simulink model "sampleModel106"  (R2022a)
settings: Solver=VariableStepAuto  StartTime=0.0  StopTime=10.0  RelTol=1e-3
undefined symbols (not defined in the file): DiscIntNeverNeededParam, magnitude, Newton, Raphson
libraries: simulink x379, slpidlib x89
(part 15 of 16)

== system sampleModel106/cfblk86/cfblk11/cfblk7/cfblk7 ==
  cfblk1 : Inport
  cfblk13 : Inport  Port=2
  cfblk14 : Inport  Port=3
  cfblk10 : Assignment  DiagnosticForDimensions=Warning  IndexOptions=Index vector (dialog)  Indices=1  OutputSizes=1
  cfblk11 : Constant  Value=[926177037.249093]  SampleTime=1
  cfblk12 : Constant  Value=[191997706.928792]  SampleTime=1
  cfblk15 : Delay
  cfblk16 : Delay
  cfblk3 : slpidlib/PID Controller (2DOF)  Controller=PID  Form=Parallel  TimeDomain=Discrete-time  UseExternalTs=off  SampleTime=-1  IntegratorMethod=Forward Euler  FilterMethod=Forward Euler  ControllerParametersSource=internal  P=1  I=1  UseKiTs=off  D=0  N=100  UseFilter=on  b=1  c=1  TunerSelectOption=Transfer Function Based (PID Tuner App)  InitialConditionSource=internal  InitialConditionForIntegrator=0  InitialConditionForFilter=0  DifferentiatorICPrevScaledInput=0  ExternalReset=none  TrackingMode=off  Kt=1  LimitOutput=off  SatLimitsSource=internal  UpperSaturationLimit=inf  LowerSaturationLimit=-inf  LinearizeAsGain=off  AntiWindupMode=none  Kb=1  POutMin=[]  POutMax=[]  IOutMin=[]  IOutMax=[]  DOutMin=[]  DOutMax=[]  NOutMin=[]  NOutMax=[]  bOutMin=[]  bOutMax=[]  cOutMin=[]  cOutMax=[]  SumOutMin=[]  SumOutMax=[]  SaturationOutMin=[]  SaturationOutMax=[]  PParamMin=[]  PParamMax=[]  IParamMin=[]  IParamMax=[]  DParamMin=[]  DParamMax=[]  NParamMin=[]  NParamMax=[]  bParamMin=[]  bParamMax=[]  cParamMin=[]  cParamMax=[]  KbParamMin=[]  KbParamMax=[]  KtParamMin=[]  KtParamMax=[]  KbOutMin=[]  KbOutMax=[]  KtOutMin=[]  KtOutMax=[]  IntegratorOutMin=[]  IntegratorOutMax=[]  FilterOutMin=[]  FilterOutMax=[]  SumI1OutMin=[]  SumI1OutMax=[]  SumI2OutMin=[]  SumI2OutMax=[]  SumI3OutMin=[]  SumI3OutMax=[]  SumI4OutMin=[]  SumI4OutMax=[]  SumDOutMin=[]  SumDOutMax=[]  Sum1OutMin=[]  Sum1OutMax=[]  Sum2OutMin=[]  Sum2OutMax=[]  Sum3OutMin=[]  Sum3OutMax=[]  DifferentiatorOutMin=[]  DifferentiatorOutMax=[]  FilterDiffOutCoefMin=[]  FilterDiffOutCoefMax=[]  ReciprocalOutMin=[]  ReciprocalOutMax=[]  SumDenOutMin=[]  SumDenOutMax=[]  SumNumOutMin=[]  SumNumOutMax=[]  DivideOutMin=[]  DivideOutMax=[]  UdiffTsProdOutMin=[]  UdiffTsProdOutMax=[]  NTsProdOutMin=[]  NTsProdOutMax=[]  UintegralTsProdOutMin=[]  UintegralTsProdOutMax=[]  UngainTsProdOutMin=[]  UngainTsProdOutMax=[]  IntegratorContinuousStateAttributes=''  IntegratorStateMustResolveToSignalObject=off  IntegratorRTWStateStorageClass=Auto  FilterContinuousStateAttributes=''  FilterStateMustResolveToSignalObject=off  FilterRTWStateStorageClass=Auto  ParallelPVariant=InternalParameters  IdealPVariant=Disabled  IVariant=InternalParameters  DVariant=InternalParameters  bVariant=InternalParameters  cVariant=InternalParameters  IntegratorVariant=Discrete  SatVariant=Disabled  AWVariant=Passthrough  PCopyVariant=Disabled  TRVariant=Disabled  FdbkBlocksVariant=Forward  IdealPFdbkVariant=Disabled  SatFdbkVariant=Disabled  DerivativeFilterVariant=ForwardEulerFilter  NVariant=InternalParameters  NCopyVariant=Disabled  FilterICVariant=InternalICsFilter  IntegratorICVariant=InternalICs  ExternalResetVariant=Disabled  TRSumVariant=Passthrough  SumFdbkVariant=Disabled  SumVariant=Sum_PID  TsampFilterVariant=InternalTs  TsampNgainVariant=Passthrough  TsampIntegralVariant=Passthrough  ExternalSaturationOutDataTypeStr=Inherit: Same as second input
      settings: SourceProductBaseCode=SL
  cfblk4 : simulink/Discrete/Transfer Fcn Real Zero  ZeroZ=0.75  ICPrevInput=0.0  DoSatur=off
      settings: SourceProductBaseCode=SL
  cfblk5 : Signum
  cfblk6 : Product
  cfblk7 : Sum  Inputs=-+
  cfblk8 : Sum  Inputs=|++
  cfblk9 : PermuteDimensions
  cfblk2 : Outport
  wires:
  cfblk1/1 -> cfblk6/1
  cfblk14/1 -> cfblk5/1
  cfblk12/1 -> cfblk8/1
  cfblk3/1 -> cfblk9/1
  cfblk11/1 -> cfblk6/2
  cfblk8/1 -> cfblk3/2, cfblk7/2
  cfblk6/1 -> cfblk2/1
  cfblk7/1 -> cfblk10/1
  cfblk4/1 -> cfblk10/2
  cfblk5/1 -> cfblk8/2
  cfblk13/1 -> cfblk7/1
  cfblk9/1 -> cfblk15/1
  cfblk15/1 -> cfblk3/1
  cfblk10/1 -> cfblk16/1
  cfblk16/1 -> cfblk4/1

== system sampleModel106/cfblk86/cfblk11/cfblk7/cfblk8 ==
  cfblk1 : Inport
  cfblk16 : Inport  Port=2
  cfblk10 : UnaryMinus
  cfblk11 : UnaryMinus
  cfblk12 : Constant  Value=[368440293.841524]  SampleTime=1
  cfblk13 : Constant  Value=[930895856.774542]  SampleTime=1
  cfblk14 : Constant  Value=[721603009.060118]  SampleTime=1
  cfblk15 : Constant  Value=[-108594991.261578]  SampleTime=1
  cfblk3 : Delay  ShowEnablePort=on
      settings: InputPortMap=u0,e6
  cfblk4 : simulink/Discrete/Tapped Delay  vinit=0.0  samptime=-1  NumDelays=1  DelayOrder=Oldest  includeCurrent=off
  cfblk5 : Sqrt  Operator=rSqrt  AlgorithmType=Newton-Raphson
  cfblk6 : Sum  Inputs=|++
  cfblk7 : Sum  Inputs=+
  cfblk8 : Squeeze
  cfblk9 : UnaryMinus
  cfblk2 : Outport
  wires:
  cfblk9/1 -> cfblk6/1
  cfblk3/1 -> cfblk5/1
  cfblk12/1 -> cfblk7/1
  cfblk15/1 -> cfblk2/1
  cfblk13/1 -> cfblk8/1
  cfblk8/1 -> cfblk6/2
  cfblk10/1 -> cfblk9/1
  cfblk16/1 -> cfblk10/1
  cfblk6/1 -> cfblk4/1
  cfblk1/1 -> cfblk11/1
  cfblk14/1 -> cfblk3/1
  cfblk7/1 -> cfblk3/2

== system sampleModel106/cfblk86/cfblk11/cfblk8/cfblk11 ==
  cfblk1 : Inport
  cfblk7 : Inport  Port=2
  cfblk3 : UnitDelay  SampleTime=-1  HasFrameUpgradeWarning=on
  cfblk4 : Constant  Value=[595381109.749089]  SampleTime=1
  cfblk5 : Constant  Value=[-747588408.733182]  SampleTime=1
  cfblk6 : Constant  Value=[-697953412.486928]  SampleTime=1
  cfblk2 : Outport
  wires:
  cfblk3/1 -> cfblk2/1
  cfblk1/1 -> cfblk3/1

== system sampleModel106/cfblk86/cfblk11/cfblk8/cfblk12 ==
  cfblk1 : Inport
  cfblk9 : Inport  Port=2
  cfblk10 : Delay
  cfblk11 : Delay
  cfblk3 : simulink/Discrete/Tapped Delay  vinit=0.0  samptime=-1  NumDelays=1  DelayOrder=Oldest  includeCurrent=off
  cfblk4 : PermuteDimensions
  cfblk5 : Math  Operator=transpose
  cfblk6 : Product  Inputs=**
  cfblk7 : DotProduct  OutDataTypeStr=Inherit: Inherit via internal rule
  cfblk8 : Constant  Value=[62268794.825662]  SampleTime=1
  cfblk2 : Outport
  wires:
  cfblk9/1 -> cfblk5/1
  cfblk7/1 -> cfblk3/1
  cfblk1/1 -> cfblk7/2
  cfblk4/1 -> cfblk6/1
  cfblk5/1 -> cfblk6/2
  cfblk8/1 -> cfblk2/1
  cfblk3/1 -> cfblk10/1
  cfblk10/1 -> cfblk7/1
  cfblk6/1 -> cfblk11/1
  cfblk11/1 -> cfblk4/1

== system sampleModel106/cfblk86/cfblk12/cfblk10/cfblk17 ==
  cfblk1 : Inport
  cfblk14 : Inport  Port=2
  Action Port : ActionPort  ActionPortLabel=if(u1 >= 0)
  cfblk10 : Product
  cfblk11 : Polyval  Coefs=[ +2.081618890e-019, -1.441693666e-014, +4.719686976e-010, -8.536869453e-006, +1.621573104e-001, -8.087801117e+001 ]
  cfblk12 : Sum  Inputs=-+
  cfblk13 : Constant  Value=[-942667236.910500]  SampleTime=1
  cfblk16 : Delay
  cfblk17 : Delay
  cfblk3 : DiscreteFir
  cfblk4 : slpidlib/PID Controller (2DOF)  Controller=PID  Form=Parallel  TimeDomain=Discrete-time  UseExternalTs=off  SampleTime=-1  IntegratorMethod=Forward Euler  FilterMethod=Forward Euler  ControllerParametersSource=internal  P=1  I=1  UseKiTs=off  D=0  N=100  UseFilter=on  b=1  c=1  TunerSelectOption=Transfer Function Based (PID Tuner App)  InitialConditionSource=internal  InitialConditionForIntegrator=0  InitialConditionForFilter=0  DifferentiatorICPrevScaledInput=0  ExternalReset=none  TrackingMode=off  Kt=1  LimitOutput=off  SatLimitsSource=internal  UpperSaturationLimit=inf  LowerSaturationLimit=-inf  LinearizeAsGain=off  AntiWindupMode=none  Kb=1  POutMin=[]  POutMax=[]  IOutMin=[]  IOutMax=[]  DOutMin=[]  DOutMax=[]  NOutMin=[]  NOutMax=[]  bOutMin=[]  bOutMax=[]  cOutMin=[]  cOutMax=[]  SumOutMin=[]  SumOutMax=[]  SaturationOutMin=[]  SaturationOutMax=[]  PParamMin=[]  PParamMax=[]  IParamMin=[]  IParamMax=[]  DParamMin=[]  DParamMax=[]  NParamMin=[]  NParamMax=[]  bParamMin=[]  bParamMax=[]  cParamMin=[]  cParamMax=[]  KbParamMin=[]  KbParamMax=[]  KtParamMin=[]  KtParamMax=[]  KbOutMin=[]  KbOutMax=[]  KtOutMin=[]  KtOutMax=[]  IntegratorOutMin=[]  IntegratorOutMax=[]  FilterOutMin=[]  FilterOutMax=[]  SumI1OutMin=[]  SumI1OutMax=[]  SumI2OutMin=[]  SumI2OutMax=[]  SumI3OutMin=[]  SumI3OutMax=[]  SumI4OutMin=[]  SumI4OutMax=[]  SumDOutMin=[]  SumDOutMax=[]  Sum1OutMin=[]  Sum1OutMax=[]  Sum2OutMin=[]  Sum2OutMax=[]  Sum3OutMin=[]  Sum3OutMax=[]  DifferentiatorOutMin=[]  DifferentiatorOutMax=[]  FilterDiffOutCoefMin=[]  FilterDiffOutCoefMax=[]  ReciprocalOutMin=[]  ReciprocalOutMax=[]  SumDenOutMin=[]  SumDenOutMax=[]  SumNumOutMin=[]  SumNumOutMax=[]  DivideOutMin=[]  DivideOutMax=[]  UdiffTsProdOutMin=[]  UdiffTsProdOutMax=[]  NTsProdOutMin=[]  NTsProdOutMax=[]  UintegralTsProdOutMin=[]  UintegralTsProdOutMax=[]  UngainTsProdOutMin=[]  UngainTsProdOutMax=[]  IntegratorContinuousStateAttributes=''  IntegratorStateMustResolveToSignalObject=off  IntegratorRTWStateStorageClass=Auto  FilterContinuousStateAttributes=''  FilterStateMustResolveToSignalObject=off  FilterRTWStateStorageClass=Auto  ParallelPVariant=InternalParameters  IdealPVariant=Disabled  IVariant=InternalParameters  DVariant=InternalParameters  bVariant=InternalParameters  cVariant=InternalParameters  IntegratorVariant=Discrete  SatVariant=Disabled  AWVariant=Passthrough  PCopyVariant=Disabled  TRVariant=Disabled  FdbkBlocksVariant=Forward  IdealPFdbkVariant=Disabled  SatFdbkVariant=Disabled  DerivativeFilterVariant=ForwardEulerFilter  NVariant=InternalParameters  NCopyVariant=Disabled  FilterICVariant=InternalICsFilter  IntegratorICVariant=InternalICs  ExternalResetVariant=Disabled  TRSumVariant=Passthrough  SumFdbkVariant=Disabled  SumVariant=Sum_PID  TsampFilterVariant=InternalTs  TsampNgainVariant=Passthrough  TsampIntegralVariant=Passthrough  ExternalSaturationOutDataTypeStr=Inherit: Same as second input
      settings: SourceProductBaseCode=SL
  cfblk5 : DiscreteIntegrator  SampleTime=-1  ICPrevOutput=DiscIntNeverNeededParam  ICPrevScaledInput=DiscIntNeverNeededParam
  cfblk6 : Sqrt  Operator=rSqrt  AlgorithmType=Newton-Raphson
  cfblk7 : Sin  TimeSource=Use external signal  SampleTime=0
  cfblk8 : Sum  Inputs=--
  cfblk9 : Rounding
  cfblk2 : Outport
  cfblk15 : Outport  Port=2
  wires:
  cfblk6/1 -> cfblk12/1
  cfblk14/1 -> cfblk6/1
  cfblk11/1 -> cfblk12/2, cfblk10/2
  cfblk9/1 -> cfblk10/1
  cfblk13/1 -> cfblk3/1
  cfblk12/1 -> cfblk8/1, cfblk17/1
  cfblk3/1 -> cfblk15/1, cfblk5/1
  cfblk8/1 -> cfblk9/1
  cfblk4/1 -> cfblk11/1
  cfblk10/1 -> cfblk7/1
  cfblk5/1 -> cfblk2/1
  cfblk1/1 -> cfblk4/1
  cfblk7/1 -> cfblk16/1
  cfblk16/1 -> cfblk8/2
  cfblk17/1 -> cfblk4/2

== system sampleModel106/cfblk86/cfblk12/cfblk10/cfblk18 ==
  cfblk1 : Inport
  cfblk10 : Inport  Port=2
  cfblk11 : Inport  Port=3
  Action Port : ActionPort  ActionPortLabel=else
  cfblk3 : Delay  DelayLengthSource=Input port
      settings: InputPortMap=u0,p1
  cfblk4 : simulink/Discrete/Tapped Delay  vinit=0.0  samptime=-1  NumDelays=1  DelayOrder=Oldest  includeCurrent=off
  cfblk5 : DotProduct  OutDataTypeStr=Inherit: Inherit via internal rule
  cfblk6 : Squeeze
  cfblk7 : Constant  Value=[600315880.016551]  SampleTime=1
  cfblk8 : Constant  Value=[-855675458.268582]  SampleTime=1
  cfblk9 : Constant  Value=[266092827.562817]  SampleTime=1
  cfblk2 : Outport
  cfblk12 : Outport  Port=2
  wires:
  cfblk3/1 -> cfblk5/1
  cfblk9/1 -> cfblk5/2
  cfblk10/1 -> cfblk4/1
  cfblk6/1 -> cfblk12/1
  cfblk8/1 -> cfblk3/1
  cfblk5/1 -> cfblk2/1
  cfblk1/1 -> cfblk3/2
  cfblk11/1 -> cfblk6/1

== system sampleModel106/cfblk86/cfblk12/cfblk11/cfblk10 ==
  cfblk1 : Inport
  cfblk11 : Inport  Port=2
  cfblk12 : Inport  Port=3
  cfblk13 : Inport  Port=4
  cfblk14 : Inport  Port=5
  cfblk10 : Constant  Value=[814482863.956402]  SampleTime=1
  cfblk3 : DiscreteStateSpace  SampleTime=-1
  cfblk4 : ComplexToRealImag
  cfblk5 : Gain  Gain=[-106543572.011716]
  cfblk6 : Signum
  cfblk7 : Abs  SaturateOnIntegerOverflow=off
  cfblk8 : Constant  Value=[-718916062.410219]  SampleTime=1
  cfblk9 : Constant  Value=[-797646911.590380]  SampleTime=1
  cfblk2 : Outport
  cfblk15 : Outport  Port=2
  wires:
  cfblk11/1 -> cfblk3/1
  cfblk13/1 -> cfblk15/1
  cfblk10/1 -> cfblk2/1
  cfblk4/1 -> cfblk5/1
  cfblk14/1 -> cfblk6/1
  cfblk3/1 -> cfblk4/1
  cfblk5/1 -> cfblk7/1

== system sampleModel106/cfblk86/cfblk12/cfblk11/cfblk11 ==
  cfblk1 : Inport
  cfblk10 : Inport  Port=2
  cfblk3 : simulink/Discrete/Transfer Fcn Real Zero  ZeroZ=0.75  ICPrevInput=0.0  DoSatur=off
      settings: SourceProductBaseCode=SL
  cfblk4 : UnitDelay  SampleTime=-1  HasFrameUpgradeWarning=on
  cfblk5 : Sum  Inputs=|++
  cfblk6 : PermuteDimensions
  cfblk7 : Gain  Gain=[693347693.453758]
  cfblk8 : Sum  Inputs=+
  cfblk9 : Gain  Gain=[980910987.680085]
  cfblk2 : Outport
  cfblk11 : Outport  Port=2
  cfblk12 : Outport  Port=3
  cfblk13 : Outport  Port=4
  wires:
  cfblk10/1 -> cfblk6/1, cfblk3/1
  cfblk9/1 -> cfblk11/1
  cfblk4/1 -> cfblk7/1
  cfblk1/1 -> cfblk8/1, cfblk2/1
  cfblk8/1 -> cfblk5/1, cfblk12/1
  cfblk5/1 -> cfblk9/1
  cfblk3/1 -> cfblk4/1
  cfblk6/1 -> cfblk5/2
  cfblk7/1 -> cfblk13/1

== system sampleModel106/cfblk86/cfblk12/cfblk11/cfblk12 ==
  cfblk1 : Inport
  cfblk13 : Inport  Port=2
  cfblk14 : Inport  Port=3
  cfblk10 : Gain  Gain=[-17064317.644250]
  cfblk11 : Abs  SaturateOnIntegerOverflow=off
  cfblk12 : Gain  Gain=[-145283411.917414]
  cfblk{16..19} (4 alike) : Delay
  cfblk3 : simulink/Discrete/Tapped Delay  vinit=0.0  samptime=-1  NumDelays=1  DelayOrder=Oldest  includeCurrent=off
  cfblk4 : Delay  ShowEnablePort=on
      settings: InputPortMap=u0,e6
  cfblk5 : Delay  DelayLengthSource=Input port
      settings: InputPortMap=u0,p1
  cfblk6 : slpidlib/PID Controller (2DOF)  Controller=PID  Form=Parallel  TimeDomain=Discrete-time  UseExternalTs=off  SampleTime=-1  IntegratorMethod=Forward Euler  FilterMethod=Forward Euler  ControllerParametersSource=internal  P=1  I=1  UseKiTs=off  D=0  N=100  UseFilter=on  b=1  c=1  TunerSelectOption=Transfer Function Based (PID Tuner App)  InitialConditionSource=internal  InitialConditionForIntegrator=0  InitialConditionForFilter=0  DifferentiatorICPrevScaledInput=0  ExternalReset=none  TrackingMode=off  Kt=1  LimitOutput=off  SatLimitsSource=internal  UpperSaturationLimit=inf  LowerSaturationLimit=-inf  LinearizeAsGain=off  AntiWindupMode=none  Kb=1  POutMin=[]  POutMax=[]  IOutMin=[]  IOutMax=[]  DOutMin=[]  DOutMax=[]  NOutMin=[]  NOutMax=[]  bOutMin=[]  bOutMax=[]  cOutMin=[]  cOutMax=[]  SumOutMin=[]  SumOutMax=[]  SaturationOutMin=[]  SaturationOutMax=[]  PParamMin=[]  PParamMax=[]  IParamMin=[]  IParamMax=[]  DParamMin=[]  DParamMax=[]  NParamMin=[]  NParamMax=[]  bParamMin=[]  bParamMax=[]  cParamMin=[]  cParamMax=[]  KbParamMin=[]  KbParamMax=[]  KtParamMin=[]  KtParamMax=[]  KbOutMin=[]  KbOutMax=[]  KtOutMin=[]  KtOutMax=[]  IntegratorOutMin=[]  IntegratorOutMax=[]  FilterOutMin=[]  FilterOutMax=[]  SumI1OutMin=[]  SumI1OutMax=[]  SumI2OutMin=[]  SumI2OutMax=[]  SumI3OutMin=[]  SumI3OutMax=[]  SumI4OutMin=[]  SumI4OutMax=[]  SumDOutMin=[]  SumDOutMax=[]  Sum1OutMin=[]  Sum1OutMax=[]  Sum2OutMin=[]  Sum2OutMax=[]  Sum3OutMin=[]  Sum3OutMax=[]  DifferentiatorOutMin=[]  DifferentiatorOutMax=[]  FilterDiffOutCoefMin=[]  FilterDiffOutCoefMax=[]  ReciprocalOutMin=[]  ReciprocalOutMax=[]  SumDenOutMin=[]  SumDenOutMax=[]  SumNumOutMin=[]  SumNumOutMax=[]  DivideOutMin=[]  DivideOutMax=[]  UdiffTsProdOutMin=[]  UdiffTsProdOutMax=[]  NTsProdOutMin=[]  NTsProdOutMax=[]  UintegralTsProdOutMin=[]  UintegralTsProdOutMax=[]  UngainTsProdOutMin=[]  UngainTsProdOutMax=[]  IntegratorContinuousStateAttributes=''  IntegratorStateMustResolveToSignalObject=off  IntegratorRTWStateStorageClass=Auto  FilterContinuousStateAttributes=''  FilterStateMustResolveToSignalObject=off  FilterRTWStateStorageClass=Auto  ParallelPVariant=InternalParameters  IdealPVariant=Disabled  IVariant=InternalParameters  DVariant=InternalParameters  bVariant=InternalParameters  cVariant=InternalParameters  IntegratorVariant=Discrete  SatVariant=Disabled  AWVariant=Passthrough  PCopyVariant=Disabled  TRVariant=Disabled  FdbkBlocksVariant=Forward  IdealPFdbkVariant=Disabled  SatFdbkVariant=Disabled  DerivativeFilterVariant=ForwardEulerFilter  NVariant=InternalParameters  NCopyVariant=Disabled  FilterICVariant=InternalICsFilter  IntegratorICVariant=InternalICs  ExternalResetVariant=Disabled  TRSumVariant=Passthrough  SumFdbkVariant=Disabled  SumVariant=Sum_PID  TsampFilterVariant=InternalTs  TsampNgainVariant=Passthrough  TsampIntegralVariant=Passthrough  ExternalSaturationOutDataTypeStr=Inherit: Same as second input
      settings: SourceProductBaseCode=SL
  cfblk7 : Sum  Inputs=|++
  cfblk8 : MinMax
  cfblk9 : Sqrt  Operator=rSqrt  AlgorithmType=Newton-Raphson
  cfblk2 : Outport
  cfblk15 : Outport  Port=2
  wires:
  cfblk1/1 -> cfblk15/1
  cfblk4/1 -> cfblk10/1
  cfblk3/1 -> cfblk6/1
  cfblk13/1 -> cfblk11/1
  cfblk12/1 -> cfblk6/2, cfblk5/1
  cfblk9/1 -> cfblk8/1, cfblk19/1
  cfblk11/1 -> cfblk12/1
  cfblk5/1 -> cfblk7/1
  cfblk6/1 -> cfblk2/1, cfblk16/1
  cfblk7/1 -> cfblk9/1
  cfblk14/1 -> cfblk4/2
  cfblk16/1 -> cfblk3/1
  cfblk10/1 -> cfblk17/1
  cfblk17/1 -> cfblk4/1
  cfblk8/1 -> cfblk18/1
  cfblk18/1 -> cfblk7/2
  cfblk19/1 -> cfblk5/2

== system sampleModel106/cfblk86/cfblk12/cfblk6/cfblk6 ==
  cfblk1 : Inport
  cfblk3 : simulink/Discrete/Transfer Fcn Lead or Lag  PoleZ=0.95  ZeroZ=0.75  ICPrevOutput=0.0  ICPrevInput=0.0  DoSatur=off
      settings: SourceProductBaseCode=SL
  cfblk4 : Reshape
  cfblk5 : Squeeze
  cfblk6 : Constant  Value=[-595129306.114251]  SampleTime=1
  cfblk7 : Constant  Value=[616259366.976854]  SampleTime=1
  cfblk8 : Constant  Value=[-570551448.739363]  SampleTime=1
  cfblk2 : Outport
  wires:
  cfblk7/1 -> cfblk3/1
  cfblk8/1 -> cfblk2/1
  cfblk6/1 -> cfblk5/1
  cfblk5/1 -> cfblk4/1

== system sampleModel106/cfblk86/cfblk12/cfblk6/cfblk7 ==
  cfblk1 : Inport
  cfblk7 : Inport  Port=2
  cfblk8 : Inport  Port=3
  cfblk12 : Delay
  cfblk3 : DiscreteTransferFcn
  cfblk4 : Assignment  DiagnosticForDimensions=Warning  IndexOptions=Index vector (dialog)  Indices=1  OutputSizes=1
  cfblk5 : Sqrt  Operator=rSqrt  AlgorithmType=Newton-Raphson
  cfblk6 : Constant  Value=[325301502.909390]  SampleTime=1
  cfblk2 : Outport
  cfblk9 : Outport  Port=2
  cfblk10 : Outport  Port=3
  cfblk11 : Outport  Port=4
  wires:
  cfblk6/1 -> cfblk2/1
  cfblk8/1 -> cfblk9/1
  cfblk1/1 -> cfblk10/1
  cfblk7/1 -> cfblk4/1
  cfblk3/1 -> cfblk5/1
  cfblk4/1 -> cfblk11/1, cfblk12/1
  cfblk5/1 -> cfblk4/2
  cfblk12/1 -> cfblk3/1

== system sampleModel106/cfblk86/cfblk12/cfblk6/cfblk8 ==
  cfblk1 : Inport
  cfblk10 : Delay
  cfblk3 : simulink/Discrete/Transfer Fcn First Order  PoleZ=0.95  ICPrevOutput=0.0  DoSatur=off
  cfblk4 : Product  Inputs=*
  cfblk5 : Rounding
  cfblk6 : Product  Inputs=*
  cfblk7 : Constant  Value=[387925012.139757]  SampleTime=1
  cfblk2 : Outport
  cfblk8 : Outport  Port=2
  cfblk9 : Outport  Port=3
  wires:
  cfblk4/1 -> cfblk5/1
  cfblk3/1 -> cfblk6/1
  cfblk5/1 -> cfblk8/1, cfblk2/1
  cfblk7/1 -> cfblk9/1
  cfblk1/1 -> cfblk4/1
  cfblk6/1 -> cfblk10/1
  cfblk10/1 -> cfblk3/1

== system sampleModel106/cfblk86/cfblk12/cfblk6/cfblk9 ==
  cfblk1 : Inport
  cfblk7 : Inport  Port=2
  cfblk8 : Inport  Port=3
  cfblk9 : Inport  Port=4
  cfblk3 : DiscreteTransferFcn
  cfblk4 : Bias  Bias=[399680849.594782]  SaturateOnIntegerOverflow=off
  cfblk5 : Constant  Value=[-667207257.082441]  SampleTime=1
  cfblk6 : Constant  Value=[329987459.255104]  SampleTime=1
  cfblk2 : Outport
  cfblk10 : Outport  Port=2
  wires:
  cfblk5/1 -> cfblk4/1
  cfblk6/1 -> cfblk10/1
  cfblk8/1 -> cfblk2/1
  cfblk1/1 -> cfblk3/1

== system sampleModel106/cfblk86/cfblk12/cfblk7/cfblk7 ==
  cfblk1 : Inport
  cfblk12 : Inport  Port=2
  cfblk13 : Inport  Port=3
  cfblk14 : Inport  Port=4
  cfblk10 : Constant  Value=[-241295018.099493]  SampleTime=1
  cfblk11 : Constant  Value=[926092452.295912]  SampleTime=1
  cfblk3 : DiscreteIntegrator  SampleTime=-1  ICPrevOutput=DiscIntNeverNeededParam  ICPrevScaledInput=DiscIntNeverNeededParam
  cfblk4 : Product  Inputs=*
  cfblk5 : simulink/Math Operations/MinMax Running Resettable  Function=min  vinit=0.0
  cfblk6 : Sum  Inputs=+-
  cfblk7 : Polyval  Coefs=[ +2.081618890e-019, -1.441693666e-014, +4.719686976e-010, -8.536869453e-006, +1.621573104e-001, -8.087801117e+001 ]
  cfblk8 : ComplexToRealImag
  cfblk9 : Constant  Value=[-944350246.390381]  SampleTime=1
  cfblk2 : Outport
  cfblk15 : Outport  Port=2
  cfblk16 : Outport  Port=3
  wires:
  cfblk11/1 -> cfblk16/1
  cfblk12/1 -> cfblk4/1
  cfblk8/1 -> cfblk15/1
  cfblk7/1 -> cfblk5/1
  cfblk4/1 -> cfblk5/2
  cfblk5/1 -> cfblk3/1
  cfblk1/1 -> cfblk7/1
  cfblk10/1 -> cfblk2/1
  cfblk9/1 -> cfblk8/1
  cfblk13/1 -> cfblk6/1
  cfblk8/2 -> cfblk6/2

== system sampleModel106/cfblk86/cfblk12/cfblk7/cfblk8 ==
  cfblk1 : Inport
  cfblk11 : Inport  Port=2
  cfblk10 : Constant  Value=[209927963.411676]  SampleTime=1
  cfblk12 : Delay
  cfblk3 : DiscreteFir
  cfblk4 : Delay
  cfblk5 : slpidlib/PID Controller  Controller=PID  Form=Parallel  TimeDomain=Discrete-time  UseExternalTs=off  SampleTime=-1  IntegratorMethod=Forward Euler  FilterMethod=Forward Euler  ControllerParametersSource=internal  P=1  I=1  UseKiTs=off  D=0  N=100  UseFilter=on  TunerSelectOption=Transfer Function Based (PID Tuner App)  InitialConditionSource=internal  InitialConditionForIntegrator=0  InitialConditionForFilter=0  DifferentiatorICPrevScaledInput=0  ExternalReset=none  TrackingMode=off  Kt=1  LimitOutput=off  SatLimitsSource=internal  UpperSaturationLimit=inf  LowerSaturationLimit=-inf  LinearizeAsGain=off  AntiWindupMode=none  Kb=1  POutMin=[]  POutMax=[]  IOutMin=[]  IOutMax=[]  DOutMin=[]  DOutMax=[]  NOutMin=[]  NOutMax=[]  SumOutMin=[]  SumOutMax=[]  SaturationOutMin=[]  SaturationOutMax=[]  PParamMin=[]  PParamMax=[]  IParamMin=[]  IParamMax=[]  DParamMin=[]  DParamMax=[]  NParamMin=[]  NParamMax=[]  KbParamMin=[]  KbParamMax=[]  KtParamMin=[]  KtParamMax=[]  KbOutMin=[]  KbOutMax=[]  KtOutMin=[]  KtOutMax=[]  IntegratorOutMin=[]  IntegratorOutMax=[]  FilterOutMin=[]  FilterOutMax=[]  SumI1OutMin=[]  SumI1OutMax=[]  SumI2OutMin=[]  SumI2OutMax=[]  SumI3OutMin=[]  SumI3OutMax=[]  SumI4OutMin=[]  SumI4OutMax=[]  SumDOutMin=[]  SumDOutMax=[]  DifferentiatorOutMin=[]  DifferentiatorOutMax=[]  FilterDiffOutCoefMin=[]  FilterDiffOutCoefMax=[]  ReciprocalOutMin=[]  ReciprocalOutMax=[]  SumDenOutMin=[]  SumDenOutMax=[]  SumNumOutMin=[]  SumNumOutMax=[]  DivideOutMin=[]  DivideOutMax=[]  UdiffTsProdOutMin=[]  UdiffTsProdOutMax=[]  NTsProdOutMin=[]  NTsProdOutMax=[]  UintegralTsProdOutMin=[]  UintegralTsProdOutMax=[]  UngainTsProdOutMin=[]  UngainTsProdOutMax=[]  IntegratorContinuousStateAttributes=''  IntegratorStateMustResolveToSignalObject=off  IntegratorRTWStateStorageClass=Auto  FilterContinuousStateAttributes=''  FilterStateMustResolveToSignalObject=off  FilterRTWStateStorageClass=Auto  ParallelPVariant=InternalParameters  IdealPVariant=Disabled  IVariant=InternalParameters  DVariant=InternalParameters  IntegratorVariant=Discrete  SatVariant=Disabled  AWVariant=Passthrough  PCopyVariant=Disabled  TRVariant=Disabled  FdbkBlocksVariant=Forward  IdealPFdbkVariant=Disabled  SatFdbkVariant=Disabled  DerivativeFilterVariant=ForwardEulerFilter  NVariant=InternalParameters  NCopyVariant=Disabled  FilterICVariant=InternalICsFilter  IntegratorICVariant=InternalICs  ExternalResetVariant=Disabled  TRSumVariant=Passthrough  SumFdbkVariant=Disabled  SumVariant=Sum_PID  TsampFilterVariant=InternalTs  TsampNgainVariant=Passthrough  TsampIntegralVariant=Passthrough  ExternalSaturationOutDataTypeStr=Inherit: Same as second input  aMode=0
  cfblk6 : UnitDelay  SampleTime=-1  HasFrameUpgradeWarning=on
  cfblk7 : Math  Operator=square
  cfblk8 : Squeeze
  cfblk9 : Gain  Gain=[496000287.857502]
  cfblk2 : Outport
  wires:
  cfblk4/1 -> cfblk2/1
  cfblk11/1 -> cfblk4/1
  cfblk7/1 -> cfblk9/1
  cfblk9/1 -> cfblk6/1
  cfblk5/1 -> cfblk7/1
  cfblk1/1 -> cfblk3/1
  cfblk10/1 -> cfblk8/1
  cfblk6/1 -> cfblk12/1
  cfblk12/1 -> cfblk5/1

== system sampleModel106/cfblk86/cfblk12/cfblk8/cfblk10 ==
  cfblk1 : Inport
  cfblk7 : Inport  Port=2
  cfblk8 : Inport  Port=3
  cfblk9 : Inport  Port=4
  cfblk10 : Inport  Port=5
  cfblk3 : DiscreteZeroPole  Poles=[0 0.5]  Gain=1  SampleTime=-1
  cfblk4 : UnaryMinus
  cfblk5 : simulink/Math Operations/MinMax Running Resettable  Function=min  vinit=0.0
  cfblk6 : Constant  Value=[-112592748.108880]  SampleTime=1
  cfblk2 : Outport
  cfblk11 : Outport  Port=2
  cfblk12 : Outport  Port=3
  wires:
  cfblk10/1 -> cfblk5/1
  cfblk1/1 -> cfblk2/1
  cfblk3/1 -> cfblk5/2
  cfblk9/1 -> cfblk3/1
  cfblk7/1 -> cfblk4/1
  cfblk5/1 -> cfblk12/1
  cfblk6/1 -> cfblk11/1

== system sampleModel106/cfblk86/cfblk12/cfblk9/cfblk7 ==
  cfblk1 : Inport
  cfblk14 : Inport  Port=2
  cfblk15 : Inport  Port=3
  cfblk10 : Squeeze
  cfblk11 : Rounding
  cfblk12 : Assignment  DiagnosticForDimensions=Warning  IndexOptions=Index vector (dialog)  Indices=1  OutputSizes=1
  cfblk13 : Constant  Value=[-907442537.447572]  SampleTime=1
  cfblk17 : Delay
  cfblk18 : Delay
  cfblk3 : simulink/Discrete/Transfer Fcn First Order  PoleZ=0.95  ICPrevOutput=0.0  DoSatur=off
  cfblk4 : simulink/Discrete/Transfer Fcn Real Zero  ZeroZ=0.75  ICPrevInput=0.0  DoSatur=off
      settings: SourceProductBaseCode=SL
  cfblk5 : simulink/Discrete/Transfer Fcn Lead or Lag  PoleZ=0.95  ZeroZ=0.75  ICPrevOutput=0.0  ICPrevInput=0.0  DoSatur=off
      settings: SourceProductBaseCode=SL
  cfblk6 : DiscreteIntegrator  SampleTime=-1  ICPrevOutput=DiscIntNeverNeededParam  ICPrevScaledInput=DiscIntNeverNeededParam
  cfblk7 : UnaryMinus
  cfblk8 : Signum
  cfblk9 : UnaryMinus
  cfblk2 : Outport
  cfblk16 : Outport  Port=2
  wires:
  cfblk15/1 -> cfblk3/1
  cfblk9/1 -> cfblk11/1
  cfblk1/1 -> cfblk5/1
  cfblk7/1 -> cfblk9/1
  cfblk11/1 -> cfblk12/1
  cfblk13/1 -> cfblk16/1
  cfblk10/1 -> cfblk7/1
  cfblk14/1 -> cfblk12/2
  cfblk6/1 -> cfblk10/1
  cfblk3/1 -> cfblk2/1
  cfblk4/1 -> cfblk8/1
  cfblk8/1 -> cfblk17/1
  cfblk17/1 -> cfblk4/1
  cfblk12/1 -> cfblk18/1
  cfblk18/1 -> cfblk6/1

== system sampleModel106/cfblk86/cfblk13/cfblk5/cfblk11 ==
  cfblk1 : Inport
  cfblk9 : Inport  Port=2
  cfblk10 : Inport  Port=3
  cfblk3 : simulink/Discrete/Tapped Delay  vinit=0.0  samptime=-1  NumDelays=1  DelayOrder=Oldest  includeCurrent=off
  cfblk4 : simulink/Discrete/Difference  ICPrevInput=0.0  OutMin=[]  OutMax=[]  OutDataTypeStr=Inherit: Inherit via back propagation  OutDataType=fixdt(1, 16)  OutScaling=2^-10  DoSatur=off
  cfblk5 : Sum  Inputs=+-
  cfblk6 : Signum
  cfblk7 : Assignment  DiagnosticForDimensions=Warning  IndexOptions=Index vector (dialog)  Indices=1  OutputSizes=1
  cfblk8 : Constant  Value=[-38653536.370818]  SampleTime=1
  cfblk2 : Outport
  wires:
  cfblk6/1 -> cfblk2/1
  cfblk8/1 -> cfblk7/1
  cfblk3/1 -> cfblk6/1
  cfblk9/1 -> cfblk7/2
  cfblk7/1 -> cfblk3/1
  cfblk10/1 -> cfblk4/1
  cfblk1/1 -> cfblk5/1
  cfblk4/1 -> cfblk5/2

== system sampleModel106/cfblk86/cfblk13/cfblk5/cfblk12 ==
  cfblk1 : Inport
  cfblk8 : Inport  Port=2
  cfblk9 : Inport  Port=3
  cfblk3 : DiscreteIntegrator  SampleTime=-1  ICPrevOutput=DiscIntNeverNeededParam  ICPrevScaledInput=DiscIntNeverNeededParam
  cfblk4 : DiscreteFilter
  cfblk5 : DiscreteZeroPole  Poles=[0 0.5]  Gain=1  SampleTime=-1
  cfblk6 : Sum  Inputs=+
  cfblk7 : Product
  cfblk2 : Outport
  cfblk10 : Outport  Port=2
  wires:
  cfblk6/1 -> cfblk5/1
  cfblk7/1 -> cfblk4/1
  cfblk8/1 -> cfblk6/1
  cfblk9/1 -> cfblk7/1
  cfblk1/1 -> cfblk7/2
  cfblk3/1 -> cfblk2/1
  cfblk4/1 -> cfblk10/1
  cfblk5/1 -> cfblk3/1

== system sampleModel106/cfblk86/cfblk13/cfblk6/cfblk6 ==
  cfblk1 : Inport
  cfblk5 : Inport  Port=2
  cfblk3 : Constant  Value=[418017958.616079]  SampleTime=1
  cfblk4 : Constant  Value=[-669585866.180650]  SampleTime=1
  cfblk2 : Outport
  cfblk6 : Outport  Port=2
  cfblk7 : Outport  Port=3
  cfblk8 : Outport  Port=4
  wires:
  cfblk4/1 -> cfblk8/1
  cfblk3/1 -> cfblk2/1
  cfblk1/1 -> cfblk6/1
  cfblk5/1 -> cfblk7/1

== system sampleModel106/cfblk86/cfblk13/cfblk7/cfblk4 ==
  cfblk1 : Inport
  cfblk11 : Inport  Port=2
  cfblk10 : Constant  Value=[428991581.145085]  SampleTime=1
  cfblk3 : UnitDelay  SampleTime=-1  HasFrameUpgradeWarning=on
  cfblk4 : Sqrt  Operator=rSqrt  AlgorithmType=Newton-Raphson
  cfblk5 : Polyval  Coefs=[ +2.081618890e-019, -1.441693666e-014, +4.719686976e-010, -8.536869453e-006, +1.621573104e-001, -8.087801117e+001 ]
  cfblk6 : Product  Inputs=*
  cfblk7 : MinMax  Function=max  Inputs=2
  cfblk8 : Gain  Gain=[-983206417.784707]
  cfblk9 : ComplexToRealImag
  cfblk2 : Outport
  wires:
  cfblk8/1 -> cfblk9/1
  cfblk10/1 -> cfblk8/1
  cfblk3/1 -> cfblk5/1
  cfblk9/1 -> cfblk3/1
  cfblk1/1 -> cfblk6/1
  cfblk11/1 -> cfblk4/1
  cfblk4/1 -> cfblk2/1
  cfblk5/1 -> cfblk7/1
  cfblk6/1 -> cfblk7/2

== system sampleModel106/cfblk86/cfblk13/cfblk7/cfblk5 ==
  cfblk1 : Inport
  cfblk10 : Inport  Port=2
  cfblk11 : Inport  Port=3
  cfblk16 : Delay
  cfblk3 : slpidlib/PID Controller  Controller=PID  Form=Parallel  TimeDomain=Discrete-time  UseExternalTs=off  SampleTime=-1  IntegratorMethod=Forward Euler  FilterMethod=Forward Euler  ControllerParametersSource=internal  P=1  I=1  UseKiTs=off  D=0  N=100  UseFilter=on  TunerSelectOption=Transfer Function Based (PID Tuner App)  InitialConditionSource=internal  InitialConditionForIntegrator=0  InitialConditionForFilter=0  DifferentiatorICPrevScaledInput=0  ExternalReset=none  TrackingMode=off  Kt=1  LimitOutput=off  SatLimitsSource=internal  UpperSaturationLimit=inf  LowerSaturationLimit=-inf  LinearizeAsGain=off  AntiWindupMode=none  Kb=1  POutMin=[]  POutMax=[]  IOutMin=[]  IOutMax=[]  DOutMin=[]  DOutMax=[]  NOutMin=[]  NOutMax=[]  SumOutMin=[]  SumOutMax=[]  SaturationOutMin=[]  SaturationOutMax=[]  PParamMin=[]  PParamMax=[]  IParamMin=[]  IParamMax=[]  DParamMin=[]  DParamMax=[]  NParamMin=[]  NParamMax=[]  KbParamMin=[]  KbParamMax=[]  KtParamMin=[]  KtParamMax=[]  KbOutMin=[]  KbOutMax=[]  KtOutMin=[]  KtOutMax=[]  IntegratorOutMin=[]  IntegratorOutMax=[]  FilterOutMin=[]  FilterOutMax=[]  SumI1OutMin=[]  SumI1OutMax=[]  SumI2OutMin=[]  SumI2OutMax=[]  SumI3OutMin=[]  SumI3OutMax=[]  SumI4OutMin=[]  SumI4OutMax=[]  SumDOutMin=[]  SumDOutMax=[]  DifferentiatorOutMin=[]  DifferentiatorOutMax=[]  FilterDiffOutCoefMin=[]  FilterDiffOutCoefMax=[]  ReciprocalOutMin=[]  ReciprocalOutMax=[]  SumDenOutMin=[]  SumDenOutMax=[]  SumNumOutMin=[]  SumNumOutMax=[]  DivideOutMin=[]  DivideOutMax=[]  UdiffTsProdOutMin=[]  UdiffTsProdOutMax=[]  NTsProdOutMin=[]  NTsProdOutMax=[]  UintegralTsProdOutMin=[]  UintegralTsProdOutMax=[]  UngainTsProdOutMin=[]  UngainTsProdOutMax=[]  IntegratorContinuousStateAttributes=''  IntegratorStateMustResolveToSignalObject=off  IntegratorRTWStateStorageClass=Auto  FilterContinuousStateAttributes=''  FilterStateMustResolveToSignalObject=off  FilterRTWStateStorageClass=Auto  ParallelPVariant=InternalParameters  IdealPVariant=Disabled  IVariant=InternalParameters  DVariant=InternalParameters  IntegratorVariant=Discrete  SatVariant=Disabled  AWVariant=Passthrough  PCopyVariant=Disabled  TRVariant=Disabled  FdbkBlocksVariant=Forward  IdealPFdbkVariant=Disabled  SatFdbkVariant=Disabled  DerivativeFilterVariant=ForwardEulerFilter  NVariant=InternalParameters  NCopyVariant=Disabled  FilterICVariant=InternalICsFilter  IntegratorICVariant=InternalICs  ExternalResetVariant=Disabled  TRSumVariant=Passthrough  SumFdbkVariant=Disabled  SumVariant=Sum_PID  TsampFilterVariant=InternalTs  TsampNgainVariant=Passthrough  TsampIntegralVariant=Passthrough  ExternalSaturationOutDataTypeStr=Inherit: Same as second input  aMode=0
  cfblk4 : simulink/Discrete/Tapped Delay  vinit=0.0  samptime=-1  NumDelays=1  DelayOrder=Oldest  includeCurrent=off
  cfblk5 : Product
  cfblk6 : Rounding
  cfblk7 : Product
  cfblk8 : PermuteDimensions
  cfblk9 : Product  Inputs=**
  cfblk2 : Outport
  cfblk12 : Outport  Port=2
  cfblk13 : Outport  Port=3
  cfblk14 : Outport  Port=4
  cfblk15 : Outport  Port=5
  wires:
  cfblk11/1 -> cfblk12/1, cfblk4/1
  cfblk5/1 -> cfblk3/1
  cfblk8/1 -> cfblk15/1
  cfblk7/1 -> cfblk8/1
  cfblk3/1 -> cfblk14/1, cfblk16/1
  cfblk6/1 -> cfblk7/1, cfblk5/2
  cfblk4/1 -> cfblk13/1
  cfblk10/1 -> cfblk9/1, cfblk2/1
  cfblk1/1 -> cfblk9/2, cfblk6/1
  cfblk9/1 -> cfblk7/2
  cfblk16/1 -> cfblk5/1

== system sampleModel106/cfblk86/cfblk13/cfblk7/cfblk6 ==
  cfblk1 : Inport
  cfblk13 : Inport  Port=2
  cfblk10 : Abs  SaturateOnIntegerOverflow=off
  cfblk11 : Constant  Value=[-507431085.295639]  SampleTime=1
  cfblk12 : Constant  Value=[481774398.768378]  SampleTime=1
  cfblk3 : DiscreteIntegrator  SampleTime=-1  ICPrevOutput=DiscIntNeverNeededParam  ICPrevScaledInput=DiscIntNeverNeededParam
  cfblk4 : simulink/Discrete/Transfer Fcn Lead or Lag  PoleZ=0.95  ZeroZ=0.75  ICPrevOutput=0.0  ICPrevInput=0.0  DoSatur=off
      settings: SourceProductBaseCode=SL
  cfblk5 : simulink/Discrete/Tapped Delay  vinit=0.0  samptime=-1  NumDelays=1  DelayOrder=Oldest  includeCurrent=off
  cfblk6 : Delay  ShowEnablePort=on
      settings: InputPortMap=u0,e6
  cfblk7 : DiscreteStateSpace  SampleTime=-1
  cfblk8 : Reshape
  cfblk9 : Sum  Inputs=+
  cfblk2 : Outport
  cfblk14 : Outport  Port=2
  cfblk15 : Outport  Port=3
  cfblk16 : Outport  Port=4
  wires:
  cfblk11/1 -> cfblk16/1
  cfblk3/1 -> cfblk7/1
  cfblk9/1 -> cfblk10/1
  cfblk13/1 -> cfblk5/1
  cfblk7/1 -> cfblk9/1
  cfblk5/1 -> cfblk4/1
  cfblk6/1 -> cfblk8/1
  cfblk4/1 -> cfblk6/1
  cfblk8/1 -> cfblk2/1
  cfblk10/1 -> cfblk14/1
  cfblk12/1 -> cfblk15/1
  cfblk1/1 -> cfblk6/2, cfblk3/1

== system sampleModel106/cfblk86/cfblk9/cfblk8/cfblk10 ==
  cfblk1 : Inport
  cfblk9 : Inport  Port=2
  cfblk10 : Inport  Port=3
  cfblk11 : Inport  Port=4
  cfblk12 : Inport  Port=5
  cfblk3 : simulink/Discrete/Transfer Fcn Real Zero  ZeroZ=0.75  ICPrevInput=0.0  DoSatur=off
      settings: SourceProductBaseCode=SL
  cfblk4 : Product
  cfblk5 : Math  Operator=magnitude^2
  cfblk6 : Sin  TimeSource=Use external signal  SampleTime=0
  cfblk7 : Constant  Value=[124003302.676543]  SampleTime=1
  cfblk8 : Constant  Value=[284375264.677964]  SampleTime=1
  cfblk2 : Outport
  cfblk13 : Outport  Port=2
  cfblk14 : Outport  Port=3
  wires:
  cfblk6/1 -> cfblk5/1
  cfblk5/1 -> cfblk4/1
  cfblk12/1 -> cfblk14/1
  cfblk9/1 -> cfblk2/1
  cfblk11/1 -> cfblk13/1
  cfblk10/1 -> cfblk3/1
  cfblk1/1 -> cfblk6/1
  cfblk7/1 -> cfblk4/2

== system sampleModel106/cfblk86/cfblk9/cfblk8/cfblk11 ==
  cfblk1 : Inport
  cfblk11 : Inport  Port=2
  cfblk10 : Constant  Value=[703380952.355505]  SampleTime=1
  cfblk3 : simulink/Math Operations/Slider Gain  gain=1  low=0  high=2
  cfblk4 : Sin  TimeSource=Use external signal  SampleTime=0
  cfblk5 : Reshape
  cfblk6 : ComplexToMagnitudeAngle
  cfblk7 : Reshape
  cfblk8 : PermuteDimensions
  cfblk9 : ComplexToRealImag
  cfblk2 : Outport
  wires:
  cfblk4/1 -> cfblk6/1
  cfblk6/1 -> cfblk3/1
  cfblk9/1 -> cfblk4/1
  cfblk9/2 -> cfblk2/1
  cfblk6/2 -> cfblk7/1
  cfblk3/1 -> cfblk5/1
  cfblk10/1 -> cfblk8/1
  cfblk1/1 -> cfblk9/1

== system sampleModel106/cfblk86/cfblk9/cfblk8/cfblk8 ==
  cfblk1 : Inport
  cfblk6 : Inport  Port=2
  cfblk7 : Inport  Port=3
  cfblk8 : Inport  Port=4
  cfblk9 : Inport  Port=5
  cfblk10 : Inport  Port=6
  cfblk11 : Inport  Port=7
  cfblk3 : Trigonometry
  cfblk4 : simulink/Math Operations/Slider Gain  gain=1  low=0  high=2
  cfblk5 : Constant  Value=[460170371.352748]  SampleTime=1
  cfblk2 : Outport
  cfblk12 : Outport  Port=2
  wires:
  cfblk7/1 -> cfblk3/1
  cfblk5/1 -> cfblk4/1
  cfblk11/1 -> cfblk2/1
  cfblk4/1 -> cfblk12/1

== system sampleModel106/cfblk86/cfblk9/cfblk8/cfblk9 ==
  cfblk1 : Inport
  cfblk13 : Inport  Port=2
  cfblk14 : Inport  Port=3
  cfblk10 : Abs  SaturateOnIntegerOverflow=off
  cfblk11 : Constant  Value=[-813698887.925377]  SampleTime=1
  cfblk12 : Constant  Value=[162105397.072125]  SampleTime=1
  cfblk3 : DiscreteTransferFcn
  cfblk4 : simulink/Discrete/Transfer Fcn Real Zero  ZeroZ=0.75  ICPrevInput=0.0  DoSatur=off
      settings: SourceProductBaseCode=SL
  cfblk5 : simulink/Discrete/Transfer Fcn First Order  PoleZ=0.95  ICPrevOutput=0.0  DoSatur=off
  cfblk6 : DiscreteIntegrator  SampleTime=-1  ICPrevOutput=DiscIntNeverNeededParam  ICPrevScaledInput=DiscIntNeverNeededParam
  cfblk7 : DotProduct  OutDataTypeStr=Inherit: Inherit via internal rule
  cfblk8 : Abs  SaturateOnIntegerOverflow=off
  cfblk9 : Product
  cfblk2 : Outport
  cfblk15 : Outport  Port=2
  wires:
  cfblk8/1 -> cfblk6/1
  cfblk3/1 -> cfblk10/1
  cfblk12/1 -> cfblk8/1
  cfblk6/1 -> cfblk5/1
  cfblk5/1 -> cfblk9/1
  cfblk11/1 -> cfblk7/1
  cfblk7/1 -> cfblk3/1
  cfblk14/1 -> cfblk9/2
  cfblk13/1 -> cfblk4/1
  cfblk9/1 -> cfblk2/1
  cfblk1/1 -> cfblk7/2
  cfblk4/1 -> cfblk15/1

== system sampleModel106/cfblk87/cfblk7/cfblk10/cfblk5 ==
  cfblk1 : Inport
  cfblk14 : Inport  Port=2
  cfblk15 : Inport  Port=3
  cfblk10 : Product
  cfblk11 : Bias  Bias=[-235476436.165482]  SaturateOnIntegerOverflow=off
  cfblk12 : simulink/Math Operations/MinMax Running Resettable  Function=min  vinit=0.0
  cfblk13 : Sum  Inputs=+-
  cfblk18 : Delay
  cfblk3 : DiscreteTransferFcn
  cfblk4 : DiscreteFilter
  cfblk5 : simulink/Discrete/Transfer Fcn Lead or Lag  PoleZ=0.95  ZeroZ=0.75  ICPrevOutput=0.0  ICPrevInput=0.0  DoSatur=off
      settings: SourceProductBaseCode=SL
  cfblk6 : Polyval  Coefs=[ +2.081618890e-019, -1.441693666e-014, +4.719686976e-010, -8.536869453e-006, +1.621573104e-001, -8.087801117e+001 ]
  cfblk7 : Product  Inputs=**
  cfblk8 : Gain  Gain=[97526613.394867]
  cfblk9 : MinMax  Inputs=2
  cfblk2 : Outport
  cfblk16 : Outport  Port=2
  cfblk17 : Outport  Port=3
  wires:
  cfblk15/1 -> cfblk5/1
  cfblk13/1 -> cfblk16/1
  cfblk10/1 -> cfblk8/1
  cfblk4/1 -> cfblk13/1, cfblk12/1, cfblk17/1
  cfblk8/1 -> cfblk4/1
  cfblk14/1 -> cfblk10/1
  cfblk6/1 -> cfblk2/1
  cfblk5/1 -> cfblk9/1
  cfblk1/1 -> cfblk7/2, cfblk12/2
  cfblk11/1 -> cfblk10/2, cfblk6/1
  cfblk7/1 -> cfblk3/1, cfblk11/1
  cfblk12/1 -> cfblk9/2
  cfblk9/1 -> cfblk13/2
  cfblk3/1 -> cfblk18/1
  cfblk18/1 -> cfblk7/1

== system sampleModel106/cfblk87/cfblk7/cfblk11/cfblk6 ==
  cfblk1 : Inport
  cfblk3 : Sum  Inputs=+-
  cfblk4 : PermuteDimensions
  cfblk5 : Signum
  cfblk6 : ComplexToMagnitudeAngle
  cfblk7 : Gain  Gain=[382038263.769144]
  cfblk8 : Product  Inputs=**
  cfblk9 : Delay
  cfblk2 : Outport
  wires:
  cfblk3/1 -> cfblk7/1
  cfblk4/1 -> cfblk8/1
  cfblk7/1 -> cfblk8/2
  cfblk5/1 -> cfblk6/1
  cfblk8/1 -> cfblk2/1
  cfblk6/2 -> cfblk4/1
  cfblk1/1 -> cfblk3/1, cfblk3/2
  cfblk6/1 -> cfblk9/1
  cfblk9/1 -> cfblk5/1

== system sampleModel106/cfblk87/cfblk8/cfblk10/cfblk10 ==
  cfblk1 : Inport
  Action Port : ActionPort  ActionPortLabel=if(u1 >= 0)
  cfblk10 : Delay
  cfblk11 : Delay
  cfblk3 : simulink/Discrete/Transfer Fcn Real Zero  ZeroZ=0.75  ICPrevInput=0.0  DoSatur=off
      settings: SourceProductBaseCode=SL
  cfblk4 : Product  Inputs=**
  cfblk5 : ComplexToMagnitudeAngle
  cfblk6 : Math  Operator=transpose
  cfblk7 : Polyval  Coefs=[ +2.081618890e-019, -1.441693666e-014, +4.719686976e-010, -8.536869453e-006, +1.621573104e-001, -8.087801117e+001 ]
  cfblk8 : Sin  TimeSource=Use external signal  SampleTime=0
  cfblk9 : Constant  Value=[-53607053.433959]  SampleTime=1
  cfblk2 : Outport
  wires:
  cfblk5/1 -> cfblk6/1
  cfblk1/1 -> cfblk4/2
  cfblk4/1 -> cfblk3/1
  cfblk5/2 -> cfblk7/1
  cfblk9/1 -> cfblk8/1
  cfblk8/1 -> cfblk2/1
  cfblk3/1 -> cfblk10/1
  cfblk10/1 -> cfblk4/1
  cfblk7/1 -> cfblk11/1
  cfblk11/1 -> cfblk5/1

== system sampleModel106/cfblk87/cfblk8/cfblk10/cfblk11 ==
  cfblk1 : Inport
  cfblk10 : Inport  Port=2
  cfblk11 : Inport  Port=3
  Action Port : ActionPort  ActionPortLabel=else
  cfblk3 : slpidlib/PID Controller (2DOF)  Controller=PID  Form=Parallel  TimeDomain=Discrete-time  UseExternalTs=off  SampleTime=-1  IntegratorMethod=Forward Euler  FilterMethod=Forward Euler  ControllerParametersSource=internal  P=1  I=1  UseKiTs=off  D=0  N=100  UseFilter=on  b=1  c=1  TunerSelectOption=Transfer Function Based (PID Tuner App)  InitialConditionSource=internal  InitialConditionForIntegrator=0  InitialConditionForFilter=0  DifferentiatorICPrevScaledInput=0  ExternalReset=none  TrackingMode=off  Kt=1  LimitOutput=off  SatLimitsSource=internal  UpperSaturationLimit=inf  LowerSaturationLimit=-inf  LinearizeAsGain=off  AntiWindupMode=none  Kb=1  POutMin=[]  POutMax=[]  IOutMin=[]  IOutMax=[]  DOutMin=[]  DOutMax=[]  NOutMin=[]  NOutMax=[]  bOutMin=[]  bOutMax=[]  cOutMin=[]  cOutMax=[]  SumOutMin=[]  SumOutMax=[]  SaturationOutMin=[]  SaturationOutMax=[]  PParamMin=[]  PParamMax=[]  IParamMin=[]  IParamMax=[]  DParamMin=[]  DParamMax=[]  NParamMin=[]  NParamMax=[]  bParamMin=[]  bParamMax=[]  cParamMin=[]  cParamMax=[]  KbParamMin=[]  KbParamMax=[]  KtParamMin=[]  KtParamMax=[]  KbOutMin=[]  KbOutMax=[]  KtOutMin=[]  KtOutMax=[]  IntegratorOutMin=[]  IntegratorOutMax=[]  FilterOutMin=[]  FilterOutMax=[]  SumI1OutMin=[]  SumI1OutMax=[]  SumI2OutMin=[]  SumI2OutMax=[]  SumI3OutMin=[]  SumI3OutMax=[]  SumI4OutMin=[]  SumI4OutMax=[]  SumDOutMin=[]  SumDOutMax=[]  Sum1OutMin=[]  Sum1OutMax=[]  Sum2OutMin=[]  Sum2OutMax=[]  Sum3OutMin=[]  Sum3OutMax=[]  DifferentiatorOutMin=[]  DifferentiatorOutMax=[]  FilterDiffOutCoefMin=[]  FilterDiffOutCoefMax=[]  ReciprocalOutMin=[]  ReciprocalOutMax=[]  SumDenOutMin=[]  SumDenOutMax=[]  SumNumOutMin=[]  SumNumOutMax=[]  DivideOutMin=[]  DivideOutMax=[]  UdiffTsProdOutMin=[]  UdiffTsProdOutMax=[]  NTsProdOutMin=[]  NTsProdOutMax=[]  UintegralTsProdOutMin=[]  UintegralTsProdOutMax=[]  UngainTsProdOutMin=[]  UngainTsProdOutMax=[]  IntegratorContinuousStateAttributes=''  IntegratorStateMustResolveToSignalObject=off  IntegratorRTWStateStorageClass=Auto  FilterContinuousStateAttributes=''  FilterStateMustResolveToSignalObject=off  FilterRTWStateStorageClass=Auto  ParallelPVariant=InternalParameters  IdealPVariant=Disabled  IVariant=InternalParameters  DVariant=InternalParameters  bVariant=InternalParameters  cVariant=InternalParameters  IntegratorVariant=Discrete  SatVariant=Disabled  AWVariant=Passthrough  PCopyVariant=Disabled  TRVariant=Disabled  FdbkBlocksVariant=Forward  IdealPFdbkVariant=Disabled  SatFdbkVariant=Disabled  DerivativeFilterVariant=ForwardEulerFilter  NVariant=InternalParameters  NCopyVariant=Disabled  FilterICVariant=InternalICsFilter  IntegratorICVariant=InternalICs  ExternalResetVariant=Disabled  TRSumVariant=Passthrough  SumFdbkVariant=Disabled  SumVariant=Sum_PID  TsampFilterVariant=InternalTs  TsampNgainVariant=Passthrough  TsampIntegralVariant=Passthrough  ExternalSaturationOutDataTypeStr=Inherit: Same as second input
      settings: SourceProductBaseCode=SL
  cfblk4 : Bias  Bias=[-660846257.413640]  SaturateOnIntegerOverflow=off
  cfblk5 : Reshape
  cfblk6 : Squeeze
  cfblk7 : UnaryMinus
  cfblk8 : Constant  Value=[467312282.852681]  SampleTime=1
  cfblk9 : Constant  Value=[-150918569.828730]  SampleTime=1
  cfblk2 : Outport
  wires:
  cfblk10/1 -> cfblk2/1
  cfblk9/1 -> cfblk6/1
  cfblk11/1 -> cfblk5/1
  cfblk7/1 -> cfblk3/1
  cfblk8/1 -> cfblk3/2
  cfblk6/1 -> cfblk4/1
  cfblk5/1 -> cfblk7/1

== system sampleModel106/cfblk87/cfblk8/cfblk10/cfblk4 ==
  cfblk1 : Inport
  cfblk3 : simulink/Discrete/Tapped Delay  vinit=0.0  samptime=-1  NumDelays=1  DelayOrder=Oldest  includeCurrent=off
  cfblk4 : UnaryMinus
  cfblk5 : Constant  Value=[841668663.491338]  SampleTime=1
  cfblk6 : Constant  Value=[-459972061.729020]  SampleTime=1
  cfblk7 : Constant  Value=[147923451.397009]  SampleTime=1
  cfblk2 : Outport
  wires:
  cfblk4/1 -> cfblk2/1
  cfblk6/1 -> cfblk3/1
  cfblk7/1 -> cfblk4/1

== system sampleModel106/cfblk87/cfblk8/cfblk10/cfblk5 ==
  cfblk1 : Inport
  cfblk10 : Abs  SaturateOnIntegerOverflow=off
  cfblk11 : Sum  Inputs=+
  cfblk12 : Constant  Value=[-733634634.154799]  SampleTime=1
  cfblk13 : Constant  Value=[-22681094.950846]  SampleTime=1
  cfblk14 : Constant  Value=[-5564414.680226]  SampleTime=1
  cfblk3 : simulink/Discrete/Transfer Fcn Real Zero  ZeroZ=0.75  ICPrevInput=0.0  DoSatur=off
      settings: SourceProductBaseCode=SL
  cfblk4 : DiscreteStateSpace  SampleTime=-1
  cfblk5 : simulink/Discrete/Tapped Delay  vinit=0.0  samptime=-1  NumDelays=1  DelayOrder=Oldest  includeCurrent=off
  cfblk6 : simulink/Discrete/Difference  ICPrevInput=0.0  OutMin=[]  OutMax=[]  OutDataTypeStr=Inherit: Inherit via back propagation  OutDataType=fixdt(1, 16)  OutScaling=2^-10  DoSatur=off
  cfblk7 : Trigonometry
  cfblk8 : ComplexToMagnitudeAngle
  cfblk9 : ComplexToRealImag
  cfblk2 : Outport
  cfblk15 : Outport  Port=2
  wires:
  cfblk5/1 -> cfblk3/1
  cfblk14/1 -> cfblk6/1
  cfblk12/1 -> cfblk9/1
  cfblk8/1 -> cfblk10/1
  cfblk1/1 -> cfblk4/1
  cfblk3/1 -> cfblk11/1
  cfblk10/1 -> cfblk7/1
  cfblk11/1 -> cfblk2/1
  cfblk6/1 -> cfblk15/1
  cfblk13/1 -> cfblk5/1
  cfblk9/1 -> cfblk8/1

== system sampleModel106/cfblk87/cfblk8/cfblk10/cfblk8 ==
  cfblk1 : Inport
  cfblk9 : Inport  Port=2
  Action Port : ActionPort  ActionPortLabel=if(u1 >= 0)
  cfblk3 : Delay  ShowEnablePort=on
      settings: InputPortMap=u0,e6
  cfblk4 : UnaryMinus
  cfblk5 : ComplexToRealImag
  cfblk6 : Sqrt  Operator=rSqrt  AlgorithmType=Newton-Raphson
  cfblk7 : Polyval  Coefs=[ +2.081618890e-019, -1.441693666e-014, +4.719686976e-010, -8.536869453e-006, +1.621573104e-001, -8.087801117e+001 ]
  cfblk8 : Constant  Value=[-227975271.493150]  SampleTime=1
  cfblk2 : Outport
  wires:
  cfblk9/1 -> cfblk3/1
  cfblk6/1 -> cfblk2/1
  cfblk8/1 -> cfblk5/1
  cfblk3/1 -> cfblk6/1
  cfblk5/1 -> cfblk7/1
  cfblk4/1 -> cfblk3/2
  cfblk1/1 -> cfblk4/1

== system sampleModel106/cfblk87/cfblk8/cfblk10/cfblk9 ==
  cfblk1 : Inport
  cfblk14 : Inport  Port=2
  Action Port : ActionPort  ActionPortLabel=else
  cfblk10 : Constant  Value=[169011946.887298]  SampleTime=1
  cfblk11 : Constant  Value=[-125928995.674470]  SampleTime=1
  cfblk12 : Constant  Value=[-385377488.164265]  SampleTime=1
  cfblk13 : Constant  Value=[247916878.378462]  SampleTime=1
  cfblk16 : Delay
  cfblk3 : simulink/Discrete/Tapped Delay  vinit=0.0  samptime=-1  NumDelays=1  DelayOrder=Oldest  includeCurrent=off
  cfblk4 : simulink/Discrete/Transfer Fcn Lead or Lag  PoleZ=0.95  ZeroZ=0.75  ICPrevOutput=0.0  ICPrevInput=0.0  DoSatur=off
      settings: SourceProductBaseCode=SL
  cfblk5 : slpidlib/PID Controller  Controller=PID  Form=Parallel  TimeDomain=Discrete-time  UseExternalTs=off  SampleTime=-1  IntegratorMethod=Forward Euler  FilterMethod=Forward Euler  ControllerParametersSource=internal  P=1  I=1  UseKiTs=off  D=0  N=100  UseFilter=on  TunerSelectOption=Transfer Function Based (PID Tuner App)  InitialConditionSource=internal  InitialConditionForIntegrator=0  InitialConditionForFilter=0  DifferentiatorICPrevScaledInput=0  ExternalReset=none  TrackingMode=off  Kt=1  LimitOutput=off  SatLimitsSource=internal  UpperSaturationLimit=inf  LowerSaturationLimit=-inf  LinearizeAsGain=off  AntiWindupMode=none  Kb=1  POutMin=[]  POutMax=[]  IOutMin=[]  IOutMax=[]  DOutMin=[]  DOutMax=[]  NOutMin=[]  NOutMax=[]  SumOutMin=[]  SumOutMax=[]  SaturationOutMin=[]  SaturationOutMax=[]  PParamMin=[]  PParamMax=[]  IParamMin=[]  IParamMax=[]  DParamMin=[]  DParamMax=[]  NParamMin=[]  NParamMax=[]  KbParamMin=[]  KbParamMax=[]  KtParamMin=[]  KtParamMax=[]  KbOutMin=[]  KbOutMax=[]  KtOutMin=[]  KtOutMax=[]  IntegratorOutMin=[]  IntegratorOutMax=[]  FilterOutMin=[]  FilterOutMax=[]  SumI1OutMin=[]  SumI1OutMax=[]  SumI2OutMin=[]  SumI2OutMax=[]  SumI3OutMin=[]  SumI3OutMax=[]  SumI4OutMin=[]  SumI4OutMax=[]  SumDOutMin=[]  SumDOutMax=[]  DifferentiatorOutMin=[]  DifferentiatorOutMax=[]  FilterDiffOutCoefMin=[]  FilterDiffOutCoefMax=[]  ReciprocalOutMin=[]  ReciprocalOutMax=[]  SumDenOutMin=[]  SumDenOutMax=[]  SumNumOutMin=[]  SumNumOutMax=[]  DivideOutMin=[]  DivideOutMax=[]  UdiffTsProdOutMin=[]  UdiffTsProdOutMax=[]  NTsProdOutMin=[]  NTsProdOutMax=[]  UintegralTsProdOutMin=[]  UintegralTsProdOutMax=[]  UngainTsProdOutMin=[]  UngainTsProdOutMax=[]  IntegratorContinuousStateAttributes=''  IntegratorStateMustResolveToSignalObject=off  IntegratorRTWStateStorageClass=Auto  FilterContinuousStateAttributes=''  FilterStateMustResolveToSignalObject=off  FilterRTWStateStorageClass=Auto  ParallelPVariant=InternalParameters  IdealPVariant=Disabled  IVariant=InternalParameters  DVariant=InternalParameters  IntegratorVariant=Discrete  SatVariant=Disabled  AWVariant=Passthrough  PCopyVariant=Disabled  TRVariant=Disabled  FdbkBlocksVariant=Forward  IdealPFdbkVariant=Disabled  SatFdbkVariant=Disabled  DerivativeFilterVariant=ForwardEulerFilter  NVariant=InternalParameters  NCopyVariant=Disabled  FilterICVariant=InternalICsFilter  IntegratorICVariant=InternalICs  ExternalResetVariant=Disabled  TRSumVariant=Passthrough  SumFdbkVariant=Disabled  SumVariant=Sum_PID  TsampFilterVariant=InternalTs  TsampNgainVariant=Passthrough  TsampIntegralVariant=Passthrough  ExternalSaturationOutDataTypeStr=Inherit: Same as second input  aMode=0
  cfblk6 : Reshape
  cfblk7 : Sum
  cfblk8 : Product
  cfblk9 : simulink/Math Operations/MinMax Running Resettable  Function=min  vinit=0.0
  cfblk2 : Outport
  cfblk15 : Outport  Port=2
  wires:
  cfblk6/1 -> cfblk9/1
  cfblk14/1 -> cfblk6/1
  cfblk7/1 -> cfblk3/1
  cfblk13/1 -> cfblk8/1
  cfblk12/1 -> cfblk9/2
  cfblk5/1 -> cfblk2/1
  cfblk9/1 -> cfblk15/1
  cfblk1/1 -> cfblk7/1
  cfblk3/1 -> cfblk8/2
  cfblk4/1 -> cfblk5/1
  cfblk10/1 -> cfblk4/1
  cfblk8/1 -> cfblk16/1
  cfblk16/1 -> cfblk7/2
